simulink library "controllers"  (R2019b)
settings: Solver=VariableStepAuto  StartTime=0.0  StopTime=10.0  RelTol=1e-3
libraries: simulink x1
settings Model: Creator=kissd  LastModifiedBy=kissd

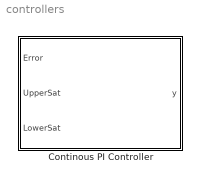
== system controllers ==
  Continous PI Controller : Subsystem  mask(Continous PI Controller){Ap=10, Ti=0.1}
      mask prompts: Ap "Proprotional Gain"; Ti "Integration Time"
      mask help: Continous PI Controller description.

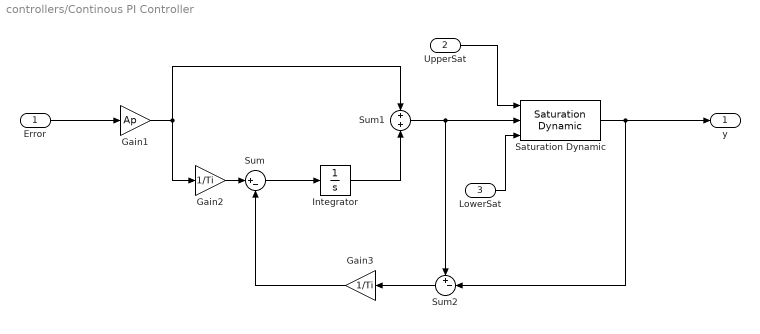
== system controllers/Continous PI Controller ==
  Error : Inport
  UpperSat : Inport  Port=2
  LowerSat : Inport  Port=3
  Gain1 : Gain  Gain=Ap
  Gain2 : Gain  Gain=1/Ti
  Gain3 : Gain  Gain=1/Ti
  Integrator : Integrator
  Saturation Dynamic : simulink/Discontinuities/Saturation Dynamic  OutMin=[]  OutMax=[]  OutDataTypeStr=Inherit: Same as second input  OutDataType=fixdt(1, 16)  OutScaling=2^-10  DoSatur=off
  Sum : Sum  Inputs=|+-
  Sum1 : Sum  Inputs=+|+
  Sum2 : Sum  Inputs=+-|
  y : Outport
  wires:
  Error/1 -> Gain1/1
  Gain2/1 -> Sum/1
  Sum/1 -> Integrator/1
  Integrator/1 -> Sum1/2
  Gain1/1 -> Gain2/1, Sum1/1
  Gain3/1 -> Sum/2
  Sum1/1 -> Saturation Dynamic/2, Sum2/1
  Saturation Dynamic/1 -> Sum2/2, y/1
  Sum2/1 -> Gain3/1
  UpperSat/1 -> Saturation Dynamic/1
  LowerSat/1 -> Saturation Dynamic/3
